simulink model "Transmission_Lines_Fault_Detection"  (R2023b)
settings: Solver=VariableStepAuto  StartTime=0.0  StopTime=0.15  RelTol=1e-3
undefined symbols (not defined in the file or in its folder): D1, Delta
libraries: spsCurrentMeasurementLib x4, spsDistributedParametersLineLib x2, spsThreePhaseVIMeasurementLib x2, spsThreePhaseParallelRLCLoadLib x1, spsThreePhaseTransformerTwoWindingsLib x1, spsThreePhaseFaultLib x1, spsThreePhaseSourceLib x1, spspowerguiLib x1
settings Model: Creator=HP  LastModifiedBy=HP

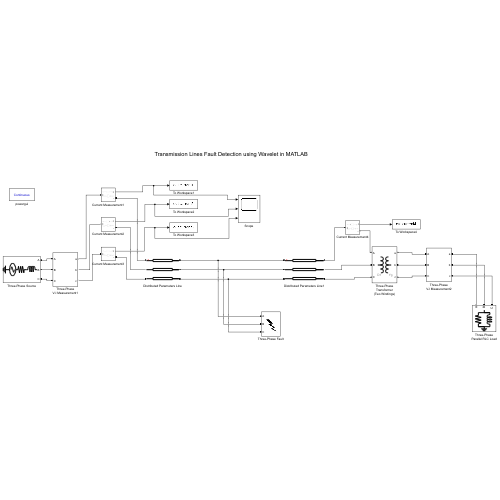
[thumbnail: Simulink's stored preview of the top-level diagram]
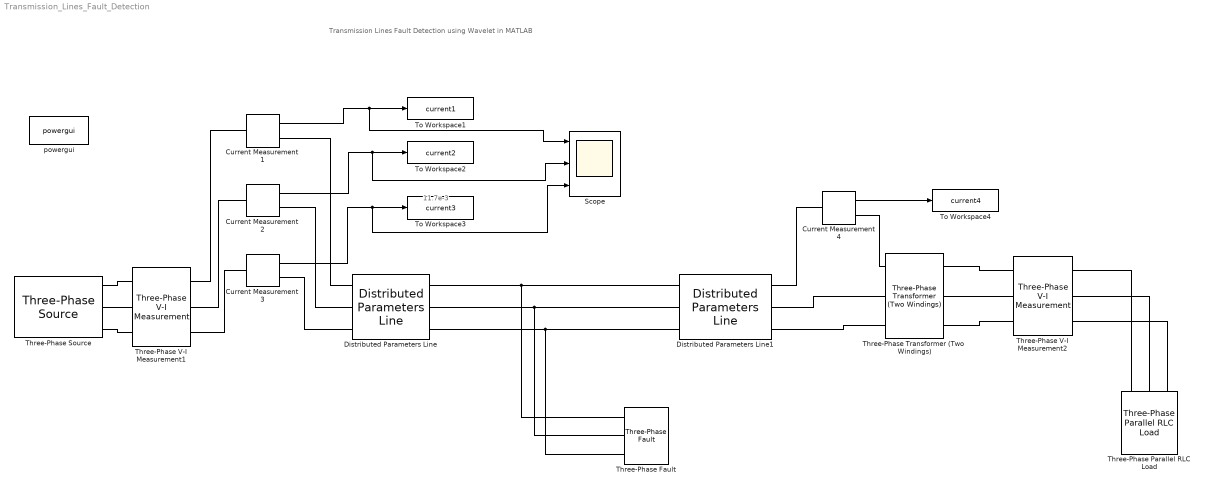
== system Transmission_Lines_Fault_Detection ==
  note: Transmission Lines Fault Detection using Wavelet in MATLAB
  note: 11.7e-3
  Current Measurement{1..4} (4 alike) : spsCurrentMeasurementLib/Current Measurement  PhasorSimulation=off  OutputType=Complex  PSBequivalent=0
  Distributed Parameters Line : spsDistributedParametersLineLib/Distributed Parameters Line  Phases=3  Length=50  Frequency=50  Resistance=[0.01273 0.3864]  Inductance="[0.9337e-3  4.1264e-3]"  Capacitance=[12.74e-9 7.751e-9]  x1=[2.5724394843075e-12 10912.2714652034 10912.2714652034;314.159265358979 314.159265358979 314.159265358979;-0.874233225006123 0.462312277142196 -1.1084840496527]  x2=[8.96901971069202e-12 10685.5908410511 10685.590841051;314.159265358979 314.159265358979 314.159265358979;-2.69870364793966 0.439349659693702 -1.13144666710119]  x3=[2.07759312832486e-13 26.711674940358 26.711674940359;314.159265358979 314.159265358979 314.159265358979;1.95504255659303 1.00491715671543 -0.565879170079437]  x4=[1.09702242958307e-13 59.1805317893529 59.1805317893527;314.159265358979 314.159265358979 314.159265358979;-1.27467400210947 0.173480669902329 -1.39731565689258]  x5=0.000282770783497871  V1=[2.572e-12 1.091e+04 1.091e+04;314.2 314.2 314.2;-0.8742 0.4623 -1.108]  V2=[8.969e-12 1.069e+04 1.069e+04;314.2 314.2 314.2;-2.699 0.4393 -1.131]  I1=[2.078e-13 26.71 26.71;314.2 314.2 314.2;1.955 1.005 -0.5659]  I2=[1.097e-13 59.18 59.18;314.2 314.2 314.2;-1.275 0.1735 -1.397]  nHarmo=1  Measurements=None  Decoupling=off  VsMag0=0  VrMag0=0  VsAngle0=0  VrAngle0=0  IsMag0=0  IrMag0=0  IsAngle0=0  IrAngle0=0
      settings: LibrarySourceBlock=sps_lib/Power Grid Elements/Distributed Parameters Line
  Distributed Parameters Line1 : spsDistributedParametersLineLib/Distributed Parameters Line  Phases=3  Length=50  Frequency=50  Resistance=[0.01273 0.3864]  Inductance="[0.9337e-3  4.1264e-3]"  Capacitance=[12.74e-9 7.751e-9]  x1=[8.96901971069202e-12 10685.5908410511 10685.590841051;314.159265358979 314.159265358979 314.159265358979;-2.69870364793966 0.439349659693702 -1.13144666710119]  x2=[1.99674999749733e-11 10433.4111825919 10433.4111825918;314.159265358979 314.159265358979 314.159265358979;-2.18442716005368 0.415478379478155 -1.15531794731674]  x3=[3.07325557597715e-13 26.7063441276429 26.7063441276431;314.159265358979 314.159265358979 314.159265358979;3.11268574710233 1.06083330674247 -0.509963020052402]  x4=[1.24511908088184e-13 59.1198595873731 59.1198595873729;314.159265358979 314.159265358979 314.159265358979;-0.116996628596567 0.119677432982981 -1.45111889381192]  x5=0.000282770783497871  V1=[8.969e-12 1.069e+04 1.069e+04;314.2 314.2 314.2;-2.699 0.4393 -1.131]  V2=[1.997e-11 1.043e+04 1.043e+04;314.2 314.2 314.2;-2.184 0.4155 -1.155]  I1=[3.073e-13 26.71 26.71;314.2 314.2 314.2;3.113 1.061 -0.51]  I2=[1.245e-13 59.12 59.12;314.2 314.2 314.2;-0.117 0.1197 -1.451]  nHarmo=1  Measurements=None  Decoupling=off  VsMag0=0  VrMag0=0  VsAngle0=0  VrAngle0=0  IsMag0=0  IrMag0=0  IsAngle0=0  IrAngle0=0
      settings: LibrarySourceBlock=sps_lib/Power Grid Elements/Distributed Parameters Line
  Scope : Scope  NumInputPorts=3
  Three-Phase Parallel RLC Load : spsThreePhaseParallelRLCLoadLib/Three-Phase Parallel RLC Load  LConnTagsString=A|B|C  Configuration=Y (grounded)  NominalVoltage=0.4e3  Vabc=[1e3 1e3 1e3]  Vabcp=[1e3 1e3 1e3]  NominalFrequency=50  UnbalancedPower=off  ActivePower=10e3  InductivePower=100  CapacitivePower=0  Pabc=[10e3 9e3 11e3]  QLabc=[100 90 110]  QCabc=[100 90 110]  Pabcp=[10e3 9e3 11e3]  QLabcp=[100 90 110]  QCabcp=[100 90 110]  Measurements=None  LoadType=constant Z
  Three-Phase Transformer (Two Windings) : spsThreePhaseTransformerTwoWindingsLib/Three-Phase Transformer (Two Windings)  Winding1Connection=Delta (D1)  Winding2Connection=Yg  CoreType=Three single-phase transformers  SetSaturation=off  Hysteresis=off  DataFile='hysteresis'  SetInitialFlux=off  Measurements=None  UNITS=pu  NominalPower=[ 100e6 , 50 ]  Winding1=[ 11e3 , 0.002 , 0.08 ]  Winding2=[0.4e3 , 0.002 , 0.08 ]  Rm=500  Lm=500  L0=0.5  Saturation=[ 0,0 ; 0.0024,1.2 ; 1.0,1.52 ]  InitialFluxes=[ 0.8 , -0.8 , 0.7 ]  BreakLoop=off  DiscreteSolver=Trapezoidal iterative  DataType=off  TransfoNumber=1
  Three-Phase V-I Measurement1 : spsThreePhaseVIMeasurementLib/Three-Phase V-I Measurement  VoltageMeasurement=phase-to-ground  SetLabelV=on  LabelV=Vabc1  Vpu=off  VpuLL=off  CurrentMeasurement=yes  SetLabelI=on  LabelI=Iabc1  Ipu=off  Pbase=100e6  Vbase=500e3  OutputType=Complex  PhasorSimulation=off  PSBequivalent=0
  Three-Phase V-I Measurement2 : spsThreePhaseVIMeasurementLib/Three-Phase V-I Measurement  VoltageMeasurement=phase-to-ground  SetLabelV=on  LabelV=Vabc2  Vpu=off  VpuLL=off  CurrentMeasurement=yes  SetLabelI=on  LabelI=Iabc2  Ipu=off  Pbase=100e6  Vbase=500e3  OutputType=Complex  PhasorSimulation=off  PSBequivalent=0
  Three-Phase Fault : spsThreePhaseFaultLib/Three-Phase Fault  InitialStates=0  FaultA=on  FaultB=off  FaultC=off  GroundFault=on  SwitchTimes="[1/50  5/50]"  External=off  SwitchStatus=NaN  FaultResistance=0.001  GroundResistance=0.01  SnubberResistance=1e6  SnubberCapacitance=inf  Measurements=None
  Three-Phase Source : spsThreePhaseSourceLib/Three-Phase Source  InternalConnection=Yg  VoltagePhases=off  Voltage=11e3  PhaseAngle=0  Voltage_phases=[25e3 25e3 25e3]/sqrt(3)  PhaseAngles_phases=[0 -120 +120]  Frequency=50  NonIdealSource=on  SpecifyImpedance=off  Resistance=0.8929  Inductance=16.58e-3  ShortCircuitLevel=100e6  BaseVoltage=11e3  XRratio=7  BusType=swing  Pref=10e3  Qref=0  Prefabc=[10e3, 10e3, 10e3]  Qrefabc=[0, 0, 0]  Qmin=-inf  Qmax=inf
  To Workspace1 : ToWorkspace  VariableName=current1  SaveFormat=Structure With Time  SampleTime=-1
  To Workspace2 : ToWorkspace  VariableName=current2  SaveFormat=Structure With Time  SampleTime=-1
  To Workspace3 : ToWorkspace  VariableName=current3  SaveFormat=Structure With Time  SampleTime=-1
  To Workspace4 : ToWorkspace  VariableName=current4  SaveFormat=Structure With Time  SampleTime=-1
  powergui : spspowerguiLib/powergui  Priority=1  SimulationMode=Continuous  SampleTime=50e-6  frequency=60  Iterations=50  frequencyindice=50  Pbase=100e6  ErrMax=1e-4  UnitsV=kV  UnitsW=MW  buscounter=0  FunctionMessages=off  echomessages=off  EnableUseOfTLC=off  CurrentSourceSwitches=on  DisableSnubberDevices=off  DisableRonSwitches=off  DisableVfSwitches=off  DisplayEquations=off  AutomaticDiscreteSolvers=off  SolverType=Tustin/Backward Euler (TBE)  Interpol=off  ExternalGateDelay=off  methode=off  Ts=100  x0status=blocks  SPID=on  SwTol=0  HookPort=off  NonlinearTolerance=1e-4  nMaxIteration=100  ContinueOnMaxIteration=off  RestoreLinks=warning  ResistiveCurrentMeasurement=off  Frange=[0:2:500]  Ylog=off  Xlog=on  ShowGrid=off  save=off  variable=ZData  structure=0  ZoomFFT=off  StartTime=0.0  cycles=1  DisplayStyle=1  fundamental=60  FreqAxis=off  MaxFrequency=1000  frequencyindicesteady=1  RmsSteady=1  display=off
  wires:
  Current Measurement1/1 -> Scope/1, To Workspace1/1
  Current Measurement2/1 -> To Workspace2/1, Scope/2
  Current Measurement3/1 -> To Workspace3/1, Scope/3
  Current Measurement4/1 -> To Workspace4/1
  connections:
  Three-Phase V-I Measurement1/LConn1 -- Three-Phase Source/RConn1
  Three-Phase Source/RConn2 -- Three-Phase V-I Measurement1/LConn2
  Three-Phase Source/RConn3 -- Three-Phase V-I Measurement1/LConn3
  Three-Phase V-I Measurement1/RConn1 -- Current Measurement1/LConn1
  Three-Phase V-I Measurement1/RConn2 -- Current Measurement2/LConn1
  Three-Phase V-I Measurement1/RConn3 -- Current Measurement3/LConn1
  Current Measurement1/RConn1 -- Distributed Parameters Line/LConn1
  Current Measurement2/RConn1 -- Distributed Parameters Line/LConn2
  Current Measurement3/RConn1 -- Distributed Parameters Line/LConn3
  Distributed Parameters Line1/RConn1 -- Current Measurement4/LConn1
  Current Measurement4/RConn1 -- Three-Phase Transformer (Two Windings)/LConn1
  Distributed Parameters Line1/RConn2 -- Three-Phase Transformer (Two Windings)/LConn2
  Distributed Parameters Line1/RConn3 -- Three-Phase Transformer (Two Windings)/LConn3
  Distributed Parameters Line/RConn1 -- Three-Phase Fault/LConn1 -- Distributed Parameters Line1/LConn1
  Distributed Parameters Line/RConn2 -- Three-Phase Fault/LConn2 -- Distributed Parameters Line1/LConn2
  Distributed Parameters Line/RConn3 -- Three-Phase Fault/LConn3 -- Distributed Parameters Line1/LConn3
  Three-Phase V-I Measurement2/LConn2 -- Three-Phase Transformer (Two Windings)/RConn2
  Three-Phase Transformer (Two Windings)/RConn3 -- Three-Phase V-I Measurement2/LConn3
  Three-Phase Transformer (Two Windings)/RConn1 -- Three-Phase V-I Measurement2/LConn1
  Three-Phase V-I Measurement2/RConn1 -- Three-Phase Parallel RLC Load/LConn1
  Three-Phase V-I Measurement2/RConn2 -- Three-Phase Parallel RLC Load/LConn2
  Three-Phase V-I Measurement2/RConn3 -- Three-Phase Parallel RLC Load/LConn3
